simulink model "Cell_model"  (R2024b)
settings: Solver=VariableStepAuto  StartTime=0.0  StopTime=1000  RelTol=1e-3
settings Model: Creator=10537  LastModifiedBy=10537

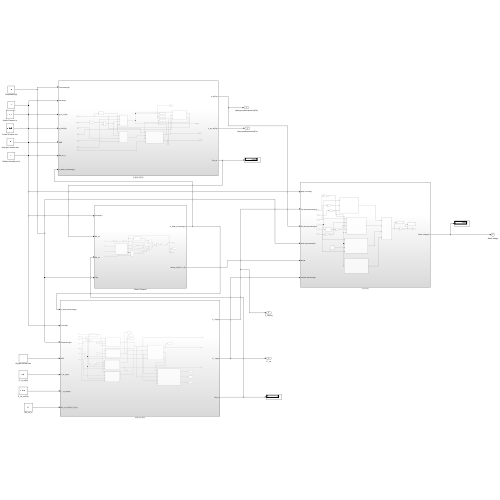
[thumbnail: Simulink's stored preview of the top-level diagram]
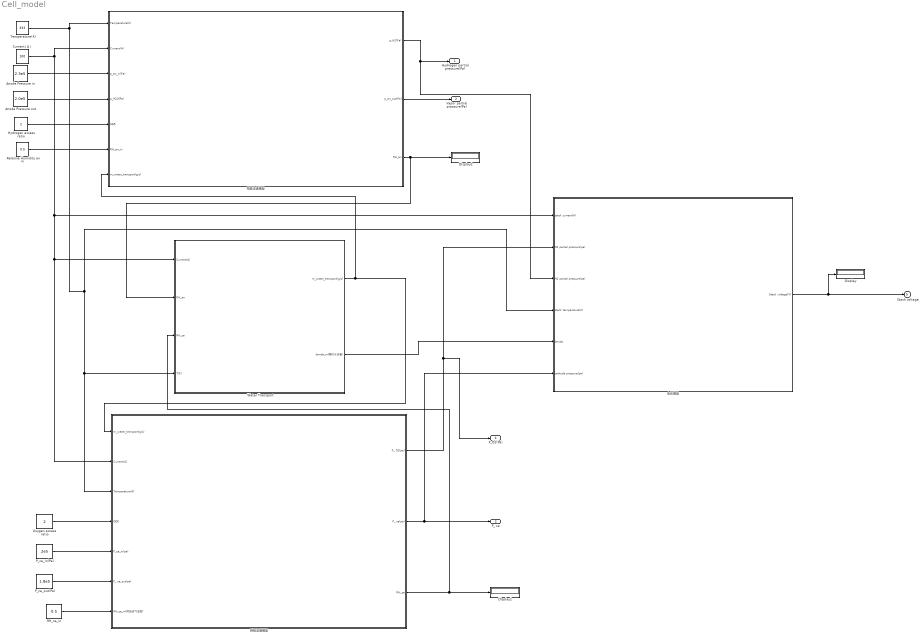
== system Cell_model ==
  " P_ca_in(Pa) " : Constant  Value=2e5
  "Anode Pressure in " : Constant  Value=2.3e5
  "Anode Pressure out " : Constant  Value=2.0e5
  "Current（A） " : Constant  Value=100
  Display : Display
  Display1 : Display
  Display2 : Display
  "Hydrogen excess ratio " : Constant  Value=2
  "Oxygen excess ratio " : Constant  Value=2
  P_ca_out(Pa) : Constant  Value=1.8e5
  RH_ca_in : Constant  Value=0.5
  Relative Humidity an in : Constant  Value=0.5
  Temperature(K) : Constant  Value=333
  Water Transport : Subsystem
  电压模型 : Subsystem
  阳极流道模型 : Subsystem
  阴极流道模型 : Subsystem
  "Hydrogen partial pressure(Pa) " : Outport  VectorParamsAs1DForOutWhenUnconnected=off
  Vapor partial pressure(Pa) : Outport  Port=2  VectorParamsAs1DForOutWhenUnconnected=off
  P_ ca : Outport  Port=3
  P_O2(Pa) : Outport  Port=4
  Stack voltage : Outport  Port=5
  wires:
  Temperature(K)/1 -> 电压模型/4(stack temperature(K)), Water Transport/4(T(K)), 阴极流道模型/3(Temperature(K)), 阳极流道模型/1(Temperature(K))
  "Current（A） "/1 -> Water Transport/1(Current(A)), 阴极流道模型/2(Current(A)), 电压模型/1(stack current(A)), 阳极流道模型/2(Current(A))
  "Anode Pressure in "/1 -> 阳极流道模型/3(p_an_in(Pa))
  "Anode Pressure out "/1 -> 阳极流道模型/4(p_H2O(Pa))
  "Hydrogen excess ratio "/1 -> 阳极流道模型/5(HER)
  Relative Humidity an in/1 -> 阳极流道模型/6(RH_an_in)
  阳极流道模型/1(p_H2(Pa)) -> 电压模型/3(H2 partial pressure(pa)), "Hydrogen partial pressure(Pa) "/1
  阳极流道模型/2(p_an_out(Pa)) -> Vapor partial pressure(Pa)/1
  "Oxygen excess ratio "/1 -> 阴极流道模型/4(OER)
  " P_ca_in(Pa) "/1 -> 阴极流道模型/5(P_ca_in(pa))
  P_ca_out(Pa)/1 -> 阴极流道模型/6(P_ ca_out(pa))
  RH_ca_in/1 -> 阴极流道模型/7(RH_ca_in(阴极进气湿度))
  阴极流道模型/1(P_ O2(pa)) -> 电压模型/2(O2 partial pressure(pa)), P_O2(Pa)/1
  阴极流道模型/2(P_ ca(pa)) -> 电压模型/6(cathode pressure(pa)), P_ ca/1
  电压模型/1(Stack voltage(V)) -> Stack voltage/1, Display/1
  阳极流道模型/3("RH_an ") -> Display2/1, Water Transport/2(RH_an)
  阴极流道模型/3(RH_ca) -> Display1/1, Water Transport/3(RH_ca)
  Water Transport/2(lamda_m(膜的水含量)) -> 电压模型/5(lamda)
  Water Transport/1(m_water_transport(g/s)) -> 阴极流道模型/1(m_water_transport(g/s)), 阳极流道模型/7(m_water_transport(g/s))

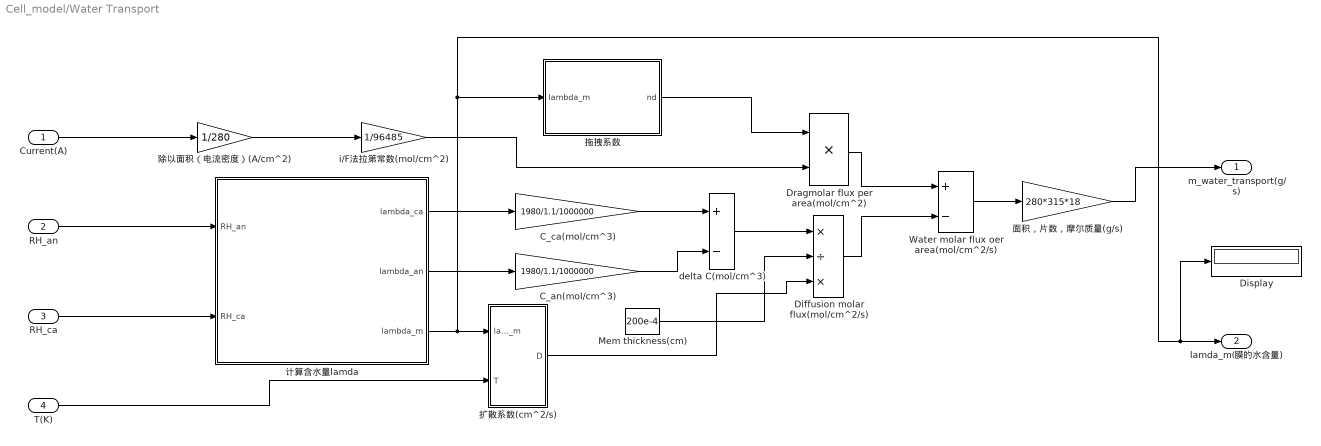
== system Cell_model/Water Transport ==
  Current(A) : Inport
  RH_an : Inport  Port=2
  RH_ca : Inport  Port=3
  T(K) : Inport  Port=4
  "\tC_an(mol/cm^3)" : Gain  Gain=1980/1.1/1000000
  "\tC_ca(mol/cm^3)" : Gain  Gain=1980/1.1/1000000
  Diffusion molar flux(mol/cm^2/s) : Product  Inputs=*/*
  Display : Display
  Dragmolar flux per area(mol/cm^2) : Product
  Mem thickness(cm) : Constant  Value=200e-4
  Water molar flux oer area(mol/cm^2/s) : Sum  Inputs=+-
  delta C(mol/cm^3) : Sum  Inputs=+-
  i/F法拉第常数(mol/cm^2) : Gain  Gain=1/96485
  扩散系数(cm^2/s) : MATLAB Function  TreatAsAtomicUnit=on
  拖拽系数 : MATLAB Function  TreatAsAtomicUnit=on
  计算含水量lamda : MATLAB Function  TreatAsAtomicUnit=on
  除以面积（电流密度）(A/cm^2) : Gain  Gain=1/280
  面积，片数，摩尔质量(g/s) : Gain  Gain=280*315*18
  m_water_transport(g/s) : Outport
  lamda_m(膜的水含量) : Outport  Port=2
  wires:
  除以面积（电流密度）(A/cm^2)/1 -> i/F法拉第常数(mol/cm^2)/1
  计算含水量lamda/1(lambda_ca) -> "\tC_ca(mol/cm^3)"/1
  计算含水量lamda/3(lambda_m) -> lamda_m(膜的水含量)/1, Display/1, 拖拽系数/1(lambda_m), 扩散系数(cm^2/s)/1(lamda_m)
  Diffusion molar flux(mol/cm^2/s)/1 -> Water molar flux oer area(mol/cm^2/s)/2
  Mem thickness(cm)/1 -> Diffusion molar flux(mol/cm^2/s)/2
  扩散系数(cm^2/s)/1(D) -> Diffusion molar flux(mol/cm^2/s)/3
  "\tC_an(mol/cm^3)"/1 -> delta C(mol/cm^3)/2
  Dragmolar flux per area(mol/cm^2)/1 -> Water molar flux oer area(mol/cm^2/s)/1
  Water molar flux oer area(mol/cm^2/s)/1 -> 面积，片数，摩尔质量(g/s)/1
  拖拽系数/1(nd) -> Dragmolar flux per area(mol/cm^2)/1
  i/F法拉第常数(mol/cm^2)/1 -> Dragmolar flux per area(mol/cm^2)/2
  delta C(mol/cm^3)/1 -> Diffusion molar flux(mol/cm^2/s)/1
  计算含水量lamda/2(lambda_an) -> "\tC_an(mol/cm^3)"/1
  "\tC_ca(mol/cm^3)"/1 -> delta C(mol/cm^3)/1
  面积，片数，摩尔质量(g/s)/1 -> m_water_transport(g/s)/1
  T(K)/1 -> 扩散系数(cm^2/s)/2(T)
  Current(A)/1 -> 除以面积（电流密度）(A/cm^2)/1
  RH_an/1 -> 计算含水量lamda/1(RH_an)
  RH_ca/1 -> 计算含水量lamda/2(RH_ca)

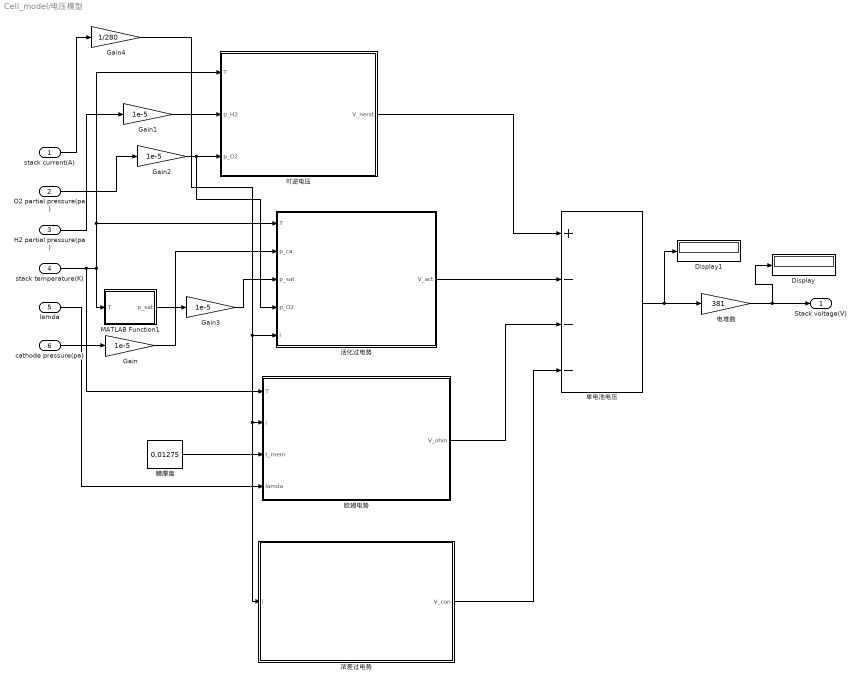
== system Cell_model/电压模型 ==
  stack current(A) : Inport
  O2 partial pressure(pa) : Inport  Port=2
  H2 partial pressure(pa) : Inport  Port=3
  stack temperature(K) : Inport  Port=4
  lamda : Inport  Port=5
  cathode pressure(pa) : Inport  Port=6
  Display : Display
  Display1 : Display
  Gain{,1..3} (4 alike) : Gain  Gain=1e-5
  Gain4 : Gain  Gain=1/280
  MATLAB Function1 : MATLAB Function  TreatAsAtomicUnit=on
  单电池电压 : Sum  Inputs=+---
  可逆电压 : MATLAB Function  TreatAsAtomicUnit=on
  欧姆电势 : MATLAB Function  TreatAsAtomicUnit=on
  活化过电势 : MATLAB Function  TreatAsAtomicUnit=on
  "浓差过电势 " : MATLAB Function  TreatAsAtomicUnit=on
  电堆数 : Gain  Gain=381
  膜厚度 : Constant  Value=0.01275
  Stack voltage(V) : Outport
  wires:
  stack temperature(K)/1 -> 欧姆电势/1(T), MATLAB Function1/1(T), 活化过电势/1(T), 可逆电压/1(T)
  O2 partial pressure(pa)/1 -> Gain2/1
  cathode pressure(pa)/1 -> Gain/1
  H2 partial pressure(pa)/1 -> Gain1/1
  膜厚度/1 -> 欧姆电势/3(t_mem)
  stack current(A)/1 -> Gain4/1
  Gain2/1 -> 活化过电势/4(p_O2), 可逆电压/3(p_O2)
  Gain4/1 -> "浓差过电势 "/1(i), 欧姆电势/2(i), 活化过电势/5(i)
  单电池电压/1 -> Display1/1, 电堆数/1
  MATLAB Function1/1(p_sat) -> Gain3/1
  Gain3/1 -> 活化过电势/3(p_sat)
  "浓差过电势 "/1(V_con) -> 单电池电压/4
  lamda/1 -> 欧姆电势/4(lamda)
  Gain/1 -> 活化过电势/2(p_ca)
  可逆电压/1(V_nerst) -> 单电池电压/1
  电堆数/1 -> Display/1, Stack voltage(V)/1
  活化过电势/1(V_act) -> 单电池电压/2
  Gain1/1 -> 可逆电压/2(p_H2)
  欧姆电势/1(V_ohm) -> 单电池电压/3

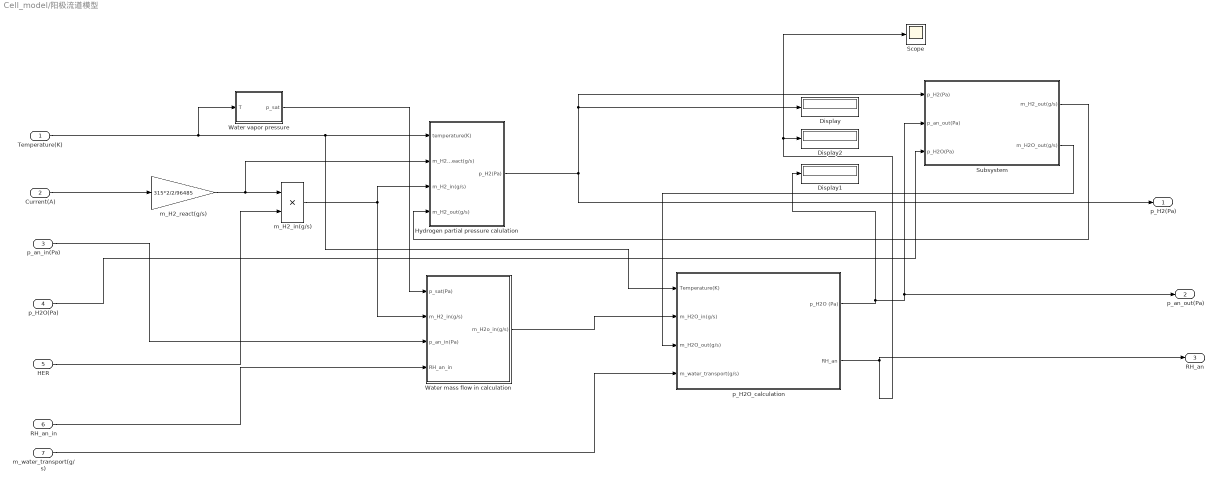
== system Cell_model/阳极流道模型 ==
  Temperature(K) : Inport
  Current(A) : Inport  Port=2
  p_an_in(Pa) : Inport  Port=3
  p_H2O(Pa) : Inport  Port=4
  HER : Inport  Port=5
  RH_an_in : Inport  Port=6
  m_water_transport(g/s) : Inport  Port=7
  Display : Display
  Display1 : Display
  Display2 : Display
  Hydrogen partial pressure calulation : Subsystem
  Scope : Scope
  Subsystem : Subsystem
  Water mass flow in calculation : Subsystem
  Water vapor pressure : MATLAB Function  TreatAsAtomicUnit=on
  m_H2_in(g/s) : Product
  m_H2_react(g/s) : Gain  Gain=315*2/2/96485
  p_H2O_calculation : Subsystem
  p_H2(Pa) : Outport
  p_an_out(Pa) : Outport  Port=2
  "RH_an " : Outport  Port=3
  wires:
  m_H2_in(g/s)/1 -> Water mass flow in calculation/2(m_H2_in(g/s)), Hydrogen partial pressure calulation/3(m_H2_in(g/s))
  Hydrogen partial pressure calulation/1(p_H2(Pa)) -> p_H2(Pa)/1, Display/1, Subsystem/1(p_H2(Pa))
  p_H2O_calculation/1(p_H2O (Pa)) -> Display1/1, p_an_out(Pa)/1, Subsystem/2(p_an_out(Pa))
  HER/1 -> m_H2_in(g/s)/2
  p_H2O_calculation/2("RH_an ") -> "RH_an "/1, Scope/1, Display2/1
  Temperature(K)/1 -> Water vapor pressure/1(T), p_H2O_calculation/1(Temperature(K)), Hydrogen partial pressure calulation/1(temperature(K))
  Subsystem/1(m_H2_out(g/s)) -> Hydrogen partial pressure calulation/4(m_H2_out(g/s))
  Subsystem/2(m_H2O_out(g/s)) -> p_H2O_calculation/3(m_H2O_out(g/s))
  m_H2_react(g/s)/1 -> Hydrogen partial pressure calulation/2(m_H2_react(g/s)), m_H2_in(g/s)/1
  Water mass flow in calculation/1(m_H2o_in(g/s)) -> p_H2O_calculation/2(m_H2O_in(g/s))
  Water vapor pressure/1(p_sat) -> Water mass flow in calculation/1(p_sat(Pa))
  p_H2O(Pa)/1 -> Subsystem/3(p_H2O(Pa))
  Current(A)/1 -> m_H2_react(g/s)/1
  RH_an_in/1 -> Water mass flow in calculation/4(RH_an_in)
  p_an_in(Pa)/1 -> Water mass flow in calculation/3(p_an_in(Pa))
  m_water_transport(g/s)/1 -> p_H2O_calculation/4(m_water_transport(g/s))

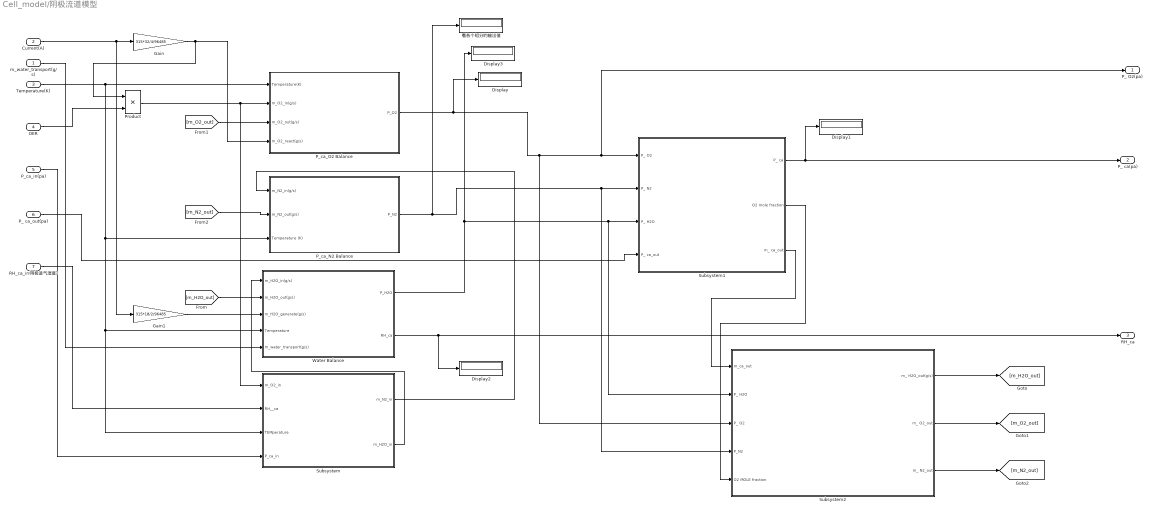
== system Cell_model/阴极流道模型 ==
  m_water_transport(g/s) : Inport
  Current(A) : Inport  Port=2
  Temperature(K) : Inport  Port=3
  OER : Inport  Port=4
  P_ca_in(pa) : Inport  Port=5
  P_ ca_out(pa) : Inport  Port=6
  RH_ca_in(阴极进气湿度) : Inport  Port=7
  Display{,1..3} (4 alike) : Display
  Gain : Gain  Gain=315*32/4/96485
  Gain1 : Gain  Gain=315*18/2/96485
  P_ca_N2 Balance : Subsystem
  P_ca_O2 Balance : Subsystem
  Product : Product
  Subsystem : Subsystem
  Subsystem1 : Subsystem
  Subsystem2 : Subsystem
  Water Balance : Subsystem
  看各个组分的输出值 : Display
  P_ O2(pa) : Outport
  P_ ca(pa) : Outport  Port=2
  RH_ca : Outport  Port=3
  wires:
  [m_H2O_out] -> Water Balance/2(m_H2O_out(g/s))
  Gain1/1 -> Water Balance/3(m_H2O_generate(g/s))
  P_ca_in(pa)/1 -> Subsystem/4(P_ca_in)
  Current(A)/1 -> Gain1/1, Gain/1
  Subsystem2/3(m_ N2_out) -> [m_N2_out]
  P_ca_N2 Balance/1(P_N2) -> 看各个组分的输出值/1, Subsystem2/4(P_N2), Subsystem1/2(P_ N2)
  Water Balance/2(RH_ca) -> RH_ca/1, Display2/1
  Subsystem/2("m_H2O_in ") -> Water Balance/1(m_H2O_in(g/s))
  Subsystem1/1(P_ ca) -> P_ ca(pa)/1, Display1/1
  Temperature(K)/1 -> Subsystem/3(TEMperature), Water Balance/4("Temperature "), P_ca_N2 Balance/3(Temperature (K)), P_ca_O2 Balance/1(Temperature(K))
  Product/1 -> Subsystem/1(m_O2_in), P_ca_O2 Balance/2(m_O2_in(g/s))
  [m_N2_out] -> P_ca_N2 Balance/2(m_N2_out(g/s))
  P_ca_O2 Balance/1(P_O2) -> Display/1, Subsystem2/3(P_ O2), P_ O2(pa)/1, Subsystem1/1(P_ O2)
  Subsystem1/2(O2 mole fraction) -> Subsystem2/5(O2 MOLE fraction)
  Subsystem/1(m_N2_in) -> P_ca_N2 Balance/1(m_N2_in(g/s))
  Subsystem2/2(m_ O2_out) -> [m_O2_out]
  Water Balance/1(P_H2O) -> Subsystem2/2(P_ H2O), Subsystem1/3(P_ H2O), Display3/1
  [m_O2_out] -> P_ca_O2 Balance/3(m_O2_out(g/s))
  P_ ca_out(pa)/1 -> Subsystem1/4(P_ ca_out)
  Gain/1 -> Product/1, P_ca_O2 Balance/4(m_O2_react(g/s))
  Subsystem1/3(m_ ca_out) -> Subsystem2/1(m_ca_out)
  Subsystem2/1(m_ H2O_out(g/s)) -> [m_H2O_out]
  OER/1 -> Product/2
  RH_ca_in(阴极进气湿度)/1 -> Subsystem/2(RH__ca)
  m_water_transport(g/s)/1 -> Water Balance/5(m_water_transport(g/s))

== system Cell_model/阳极流道模型/Hydrogen partial pressure calulation ==
  temperature(K) : Inport
  m_H2_react(g/s) : Inport  Port=2
  m_H2_in(g/s) : Inport  Port=3
  m_H2_out(g/s) : Inport  Port=4
  Gain : Gain  Gain=8.314/2/0.005
  dm_H2/dt(g/s) : Sum  Inputs=+--
  m_H2(g) : Integrator  InitialCondition=0.01
  p_H2 : Product
  p_H2(Pa) : Outport  VectorParamsAs1DForOutWhenUnconnected=off
  wires:
  m_H2_in(g/s)/1 -> dm_H2/dt(g/s)/1
  m_H2(g)/1 -> Gain/1
  m_H2_react(g/s)/1 -> dm_H2/dt(g/s)/2
  Gain/1 -> p_H2/2
  dm_H2/dt(g/s)/1 -> m_H2(g)/1
  p_H2/1 -> p_H2(Pa)/1
  m_H2_out(g/s)/1 -> dm_H2/dt(g/s)/3
  temperature(K)/1 -> p_H2/1

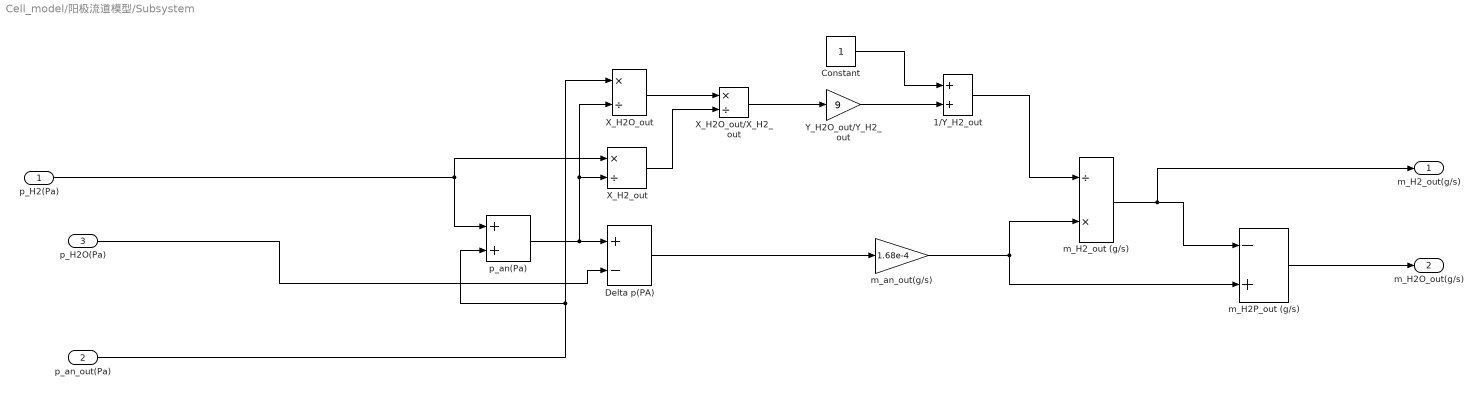
== system Cell_model/阳极流道模型/Subsystem ==
  p_H2(Pa) : Inport
  p_an_out(Pa) : Inport  Port=2
  p_H2O(Pa) : Inport  Port=3
  1/Y_H2_out : Sum
  Constant : Constant
  Delta p(PA) : Sum  Inputs=+-
  X_H2O_out : Product  Inputs=*/
  X_H2O_out/X_H2_out : Product  Inputs=*/
  X_H2_out : Product  Inputs=*/
  Y_H2O_out/Y_H2_out : Gain  Gain=9
  m_H2P_out (g/s) : Sum  Inputs=-+
  m_H2_out (g/s) : Product  Inputs=/*
  m_an_out(g/s) : Gain  Gain=1.68e-4
  p_an(Pa) : Sum
  m_H2_out(g/s) : Outport  VectorParamsAs1DForOutWhenUnconnected=off
  m_H2O_out(g/s) : Outport  Port=2  VectorParamsAs1DForOutWhenUnconnected=off
  wires:
  Delta p(PA)/1 -> m_an_out(g/s)/1
  X_H2O_out/X_H2_out/1 -> Y_H2O_out/Y_H2_out/1
  p_an(Pa)/1 -> X_H2_out/2, X_H2O_out/2, Delta p(PA)/1
  p_H2(Pa)/1 -> p_an(Pa)/1, X_H2_out/1
  m_H2_out (g/s)/1 -> m_H2_out(g/s)/1, m_H2P_out (g/s)/1
  m_an_out(g/s)/1 -> m_H2P_out (g/s)/2, m_H2_out (g/s)/2
  1/Y_H2_out/1 -> m_H2_out (g/s)/1
  p_an_out(Pa)/1 -> p_an(Pa)/2, X_H2O_out/1
  Y_H2O_out/Y_H2_out/1 -> 1/Y_H2_out/2
  Constant/1 -> 1/Y_H2_out/1
  X_H2_out/1 -> X_H2O_out/X_H2_out/2
  X_H2O_out/1 -> X_H2O_out/X_H2_out/1
  m_H2P_out (g/s)/1 -> m_H2O_out(g/s)/1
  p_H2O(Pa)/1 -> Delta p(PA)/2

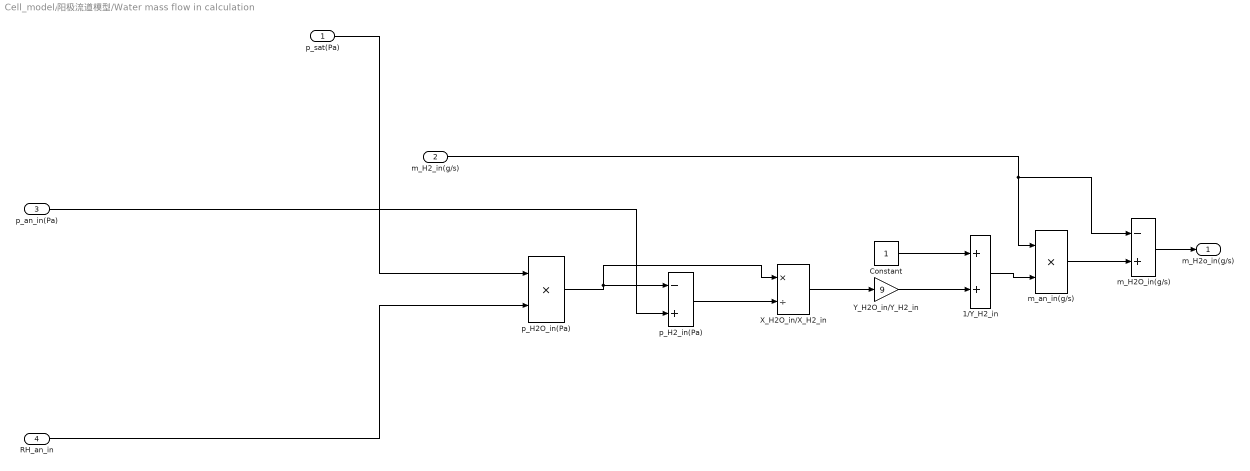
== system Cell_model/阳极流道模型/Water mass flow in calculation ==
  p_sat(Pa) : Inport
  m_H2_in(g/s) : Inport  Port=2
  p_an_in(Pa) : Inport  Port=3
  RH_an_in : Inport  Port=4
  1/Y_H2_in : Sum
  Constant : Constant
  X_H2O_in/X_H2_in : Product  Inputs=*/
  Y_H2O_in/Y_H2_in : Gain  Gain=9
  m_H2O_in(g/s) : Sum  Inputs=-+
  m_an_in(g/s) : Product
  p_H2O_in(Pa) : Product
  p_H2_in(Pa) : Sum  Inputs=-+
  m_H2o_in(g/s) : Outport  VectorParamsAs1DForOutWhenUnconnected=off
  wires:
  1/Y_H2_in/1 -> m_an_in(g/s)/2
  m_an_in(g/s)/1 -> m_H2O_in(g/s)/2
  m_H2_in(g/s)/1 -> m_an_in(g/s)/1, m_H2O_in(g/s)/1
  p_an_in(Pa)/1 -> p_H2_in(Pa)/2
  Y_H2O_in/Y_H2_in/1 -> 1/Y_H2_in/2
  X_H2O_in/X_H2_in/1 -> Y_H2O_in/Y_H2_in/1
  Constant/1 -> 1/Y_H2_in/1
  p_H2_in(Pa)/1 -> X_H2O_in/X_H2_in/2
  p_H2O_in(Pa)/1 -> X_H2O_in/X_H2_in/1, p_H2_in(Pa)/1
  m_H2O_in(g/s)/1 -> m_H2o_in(g/s)/1
  p_sat(Pa)/1 -> p_H2O_in(Pa)/1
  RH_an_in/1 -> p_H2O_in(Pa)/2

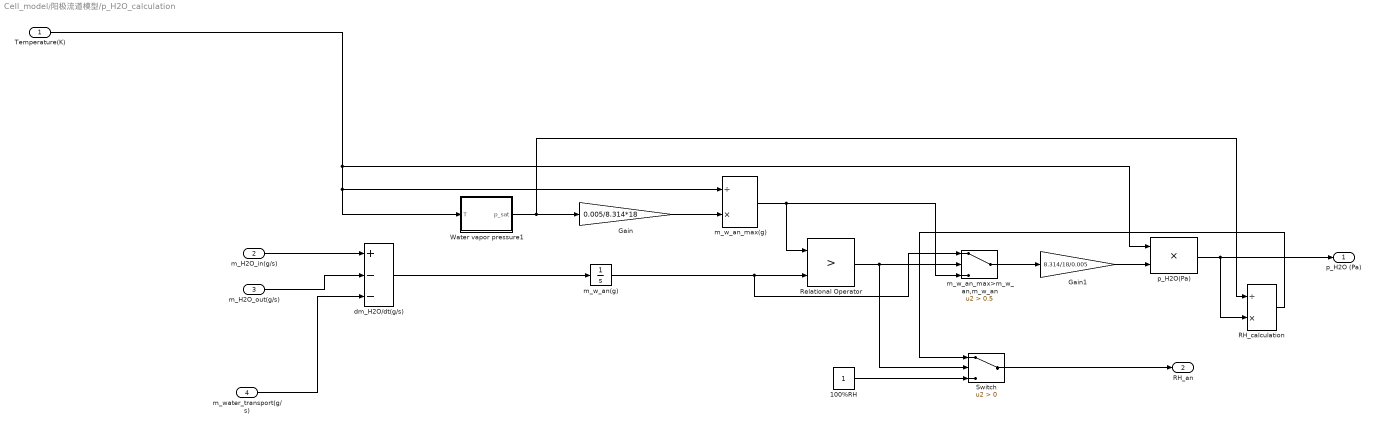
== system Cell_model/阳极流道模型/p_H2O_calculation ==
  Temperature(K) : Inport
  m_H2O_in(g/s) : Inport  Port=2
  m_H2O_out(g/s) : Inport  Port=3
  m_water_transport(g/s) : Inport  Port=4
  100%RH : Constant
  Gain : Gain  Gain=0.005/8.314*18
  Gain1 : Gain  Gain=8.314/18/0.005
  "RH_calculation " : Product  Inputs=/*
  Relational Operator : RelationalOperator  Operator=>  OutDataTypeStr=boolean  RndMeth=Simplest  InputSameDT=off
  Switch : Switch  Criteria=u2 > Threshold  SaturateOnIntegerOverflow=off  InputSameDT=off
  Water vapor pressure1 : MATLAB Function  TreatAsAtomicUnit=on
  dm_H2O/dt(g/s) : Sum  Inputs=+--
  m_w_an(g) : Integrator  InitialCondition=0.01
  m_w_an_max(g) : Product  Inputs=/*
  m_w_an_max>m_w_an,m_w_an : Switch  Criteria=u2 > Threshold  Threshold=0.5  SaturateOnIntegerOverflow=off  InputSameDT=off
  p_H2O(Pa) : Product
  p_H2O (Pa) : Outport  VectorParamsAs1DForOutWhenUnconnected=off
  "RH_an " : Outport  Port=2  VectorParamsAs1DForOutWhenUnconnected=off
  wires:
  Temperature(K)/1 -> Water vapor pressure1/1(T), m_w_an_max(g)/1, p_H2O(Pa)/1
  100%RH/1 -> Switch/3
  m_w_an_max(g)/1 -> m_w_an_max>m_w_an,m_w_an/3, Relational Operator/1
  dm_H2O/dt(g/s)/1 -> m_w_an(g)/1
  Switch/1 -> "RH_an "/1
  m_w_an(g)/1 -> m_w_an_max>m_w_an,m_w_an/1, Relational Operator/2
  Water vapor pressure1/1(p_sat) -> "RH_calculation "/1, Gain/1
  Relational Operator/1 -> Switch/2, m_w_an_max>m_w_an,m_w_an/2
  p_H2O(Pa)/1 -> p_H2O (Pa)/1, "RH_calculation "/2
  Gain1/1 -> p_H2O(Pa)/2
  m_w_an_max>m_w_an,m_w_an/1 -> Gain1/1
  "RH_calculation "/1 -> Switch/1
  Gain/1 -> m_w_an_max(g)/2
  m_H2O_out(g/s)/1 -> dm_H2O/dt(g/s)/2
  m_H2O_in(g/s)/1 -> dm_H2O/dt(g/s)/1
  m_water_transport(g/s)/1 -> dm_H2O/dt(g/s)/3

== system Cell_model/阴极流道模型/P_ca_N2 Balance ==
  m_N2_in(g/s) : Inport
  m_N2_out(g/s) : Inport  Port=2
  Temperature (K) : Inport  Port=3
  Add : Sum  Inputs=+-
  Gain1 : Gain  Gain=8.314/28/0.01
  Product1 : Product
  m_ca_N2 : Integrator  InitialCondition=0.01
  P_N2 : Outport  VectorParamsAs1DForOutWhenUnconnected=off
  wires:
  Add/1 -> m_ca_N2/1
  m_N2_in(g/s)/1 -> Add/1
  m_N2_out(g/s)/1 -> Add/2
  Temperature (K)/1 -> Product1/2
  Gain1/1 -> Product1/1
  Product1/1 -> P_N2/1
  m_ca_N2/1 -> Gain1/1

== system Cell_model/阴极流道模型/P_ca_O2 Balance ==
  Temperature(K) : Inport
  m_O2_in(g/s) : Inport  Port=2
  m_O2_out(g/s) : Inport  Port=3
  m_O2_react(g/s) : Inport  Port=4
  Add : Sum  Inputs=+--
  Gain : Gain  Gain=8.314/32/0.01
  Product : Product
  m_ca_O2 : Integrator  InitialCondition=4.2e4
  P_O2 : Outport  VectorParamsAs1DForOutWhenUnconnected=off
  wires:
  m_O2_react(g/s)/1 -> Add/3
  m_O2_in(g/s)/1 -> Add/1
  Add/1 -> Gain/1
  Temperature(K)/1 -> Product/1
  Gain/1 -> Product/2
  m_O2_out(g/s)/1 -> Add/2
  Product/1 -> m_ca_O2/1
  m_ca_O2/1 -> P_O2/1

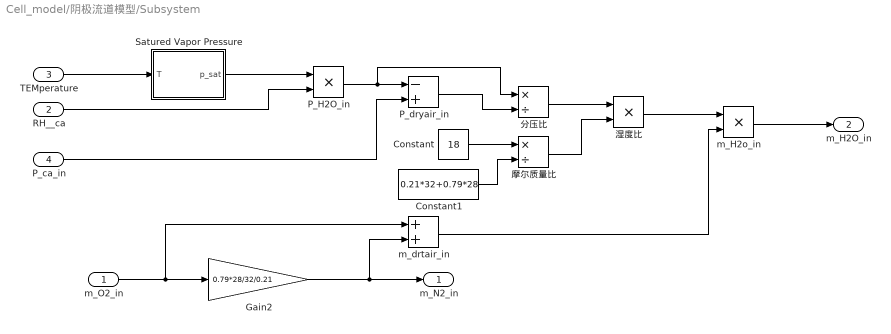
== system Cell_model/阴极流道模型/Subsystem ==
  m_O2_in : Inport
  RH__ca : Inport  Port=2
  TEMperature : Inport  Port=3
  P_ca_in : Inport  Port=4
  Constant : Constant  Value=18
  Constant1 : Constant  Value=0.21*32+0.79*28
  Gain2 : Gain  Gain=0.79*28/32/0.21
  P_H2O_in : Product
  P_dryair_in : Sum  Inputs=-+
  "Satured Vapor Pressure " : MATLAB Function  TreatAsAtomicUnit=on
  "m_H2o_in " : Product
  m_drtair_in : Sum
  分压比 : Product  Inputs=*/
  摩尔质量比 : Product  Inputs=*/
  湿度比 : Product
  m_N2_in : Outport  VectorParamsAs1DForOutWhenUnconnected=off
  "m_H2O_in " : Outport  Port=2  VectorParamsAs1DForOutWhenUnconnected=off
  wires:
  TEMperature/1 -> "Satured Vapor Pressure "/1(T)
  P_ca_in/1 -> P_dryair_in/2
  Gain2/1 -> m_N2_in/1, m_drtair_in/2
  P_H2O_in/1 -> 分压比/1, P_dryair_in/1
  m_O2_in/1 -> m_drtair_in/1, Gain2/1
  Constant1/1 -> 摩尔质量比/2
  摩尔质量比/1 -> 湿度比/2
  湿度比/1 -> "m_H2o_in "/1
  m_drtair_in/1 -> "m_H2o_in "/2
  Constant/1 -> 摩尔质量比/1
  RH__ca/1 -> P_H2O_in/2
  P_dryair_in/1 -> 分压比/2
  "Satured Vapor Pressure "/1(p_sat) -> P_H2O_in/1
  "m_H2o_in "/1 -> "m_H2O_in "/1
  分压比/1 -> 湿度比/1

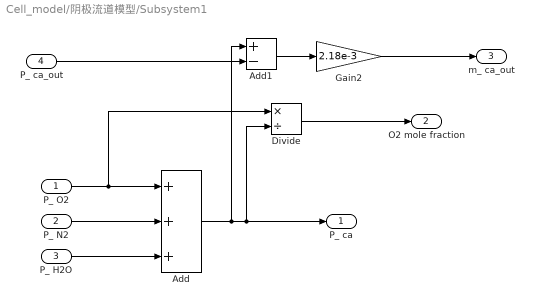
== system Cell_model/阴极流道模型/Subsystem1 ==
  P_ O2 : Inport
  P_ N2 : Inport  Port=2
  P_ H2O : Inport  Port=3
  P_ ca_out : Inport  Port=4
  Add : Sum  Inputs=+++
  Add1 : Sum  Inputs=+-
  Divide : Product  Inputs=*/
  Gain2 : Gain  Gain=2.18e-3
  P_ ca : Outport
  O2 mole fraction : Outport  Port=2
  m_ ca_out : Outport  Port=3
  wires:
  Add1/1 -> Gain2/1
  Add/1 -> Add1/1, P_ ca/1, Divide/2
  P_ H2O/1 -> Add/3
  P_ N2/1 -> Add/2
  P_ ca_out/1 -> Add1/2
  Gain2/1 -> m_ ca_out/1
  P_ O2/1 -> Divide/1, Add/1
  Divide/1 -> O2 mole fraction/1

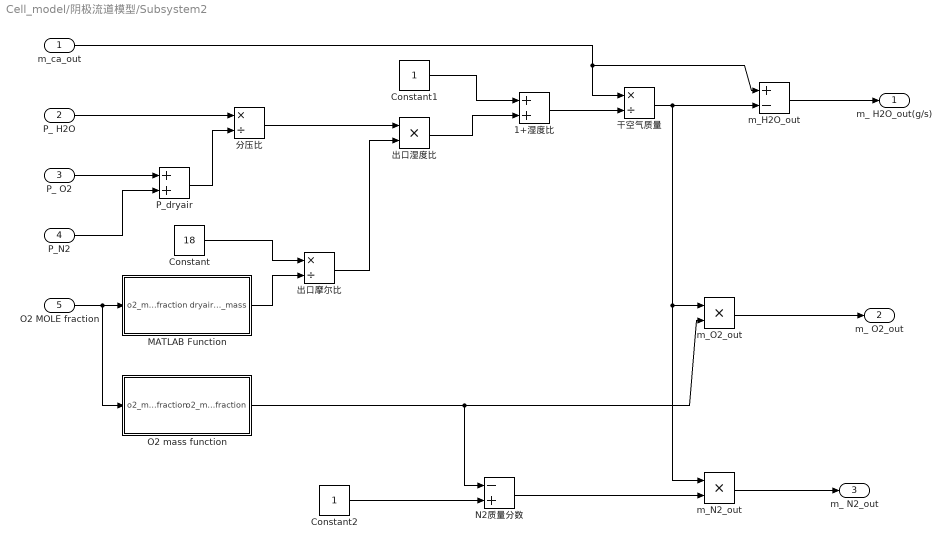
== system Cell_model/阴极流道模型/Subsystem2 ==
  m_ca_out : Inport
  P_ H2O : Inport  Port=2
  P_ O2 : Inport  Port=3
  P_N2 : Inport  Port=4
  O2 MOLE fraction : Inport  Port=5
  1+湿度比 : Sum
  Constant : Constant  Value=18
  Constant1 : Constant
  Constant2 : Constant
  MATLAB Function : MATLAB Function  TreatAsAtomicUnit=on
  N2质量分数 : Sum  Inputs=-+
  O2 mass function : MATLAB Function  TreatAsAtomicUnit=on
  P_dryair : Sum
  m_H2O_out : Sum  Inputs=+-
  m_N2_out : Product
  m_O2_out : Product
  出口摩尔比 : Product  Inputs=*/
  出口湿度比 : Product
  分压比 : Product  Inputs=*/
  干空气质量 : Product  Inputs=*/
  m_ H2O_out(g/s) : Outport
  m_ O2_out : Outport  Port=2
  m_ N2_out : Outport  Port=3
  wires:
  P_dryair/1 -> 分压比/2
  m_ca_out/1 -> m_H2O_out/1, 干空气质量/1
  m_H2O_out/1 -> m_ H2O_out(g/s)/1
  出口摩尔比/1 -> 出口湿度比/2
  出口湿度比/1 -> 1+湿度比/2
  O2 mass function/1(o2_mass_fraction) -> N2质量分数/1, m_O2_out/2
  m_O2_out/1 -> m_ O2_out/1
  干空气质量/1 -> m_H2O_out/2, m_O2_out/1, m_N2_out/1
  P_N2/1 -> P_dryair/2
  N2质量分数/1 -> m_N2_out/2
  P_ O2/1 -> P_dryair/1
  1+湿度比/1 -> 干空气质量/2
  Constant2/1 -> N2质量分数/2
  P_ H2O/1 -> 分压比/1
  分压比/1 -> 出口湿度比/1
  O2 MOLE fraction/1 -> O2 mass function/1(o2_mole_fraction), MATLAB Function/1(o2_mole_fraction)
  MATLAB Function/1(dryair_mole_mass) -> 出口摩尔比/2
  Constant/1 -> 出口摩尔比/1
  Constant1/1 -> 1+湿度比/1
  m_N2_out/1 -> m_ N2_out/1

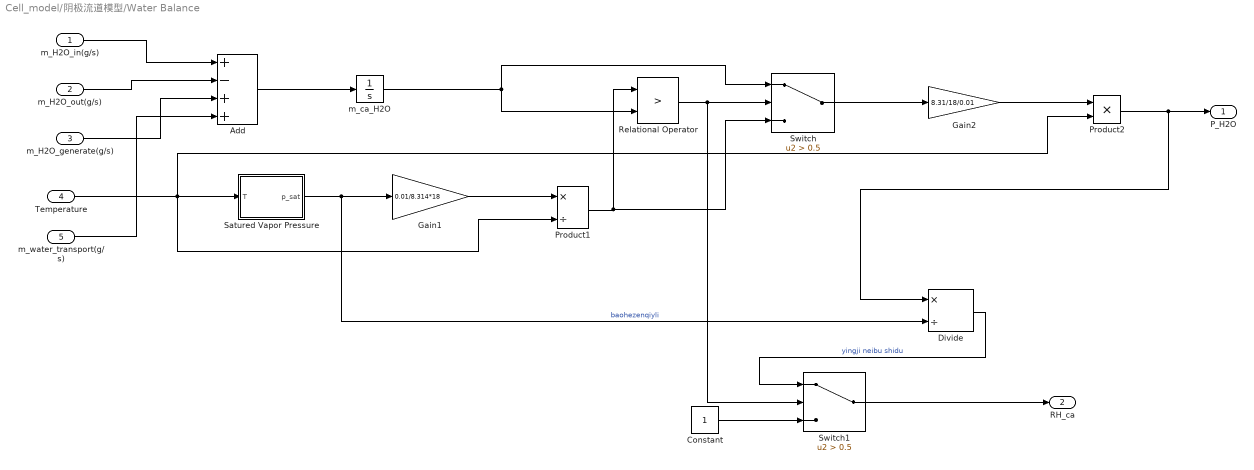
== system Cell_model/阴极流道模型/Water Balance ==
  m_H2O_in(g/s) : Inport
  m_H2O_out(g/s) : Inport  Port=2
  m_H2O_generate(g/s) : Inport  Port=3
  "Temperature " : Inport  Port=4
  m_water_transport(g/s) : Inport  Port=5
  Add : Sum  Inputs=+-++
  Constant : Constant
  Divide : Product  Inputs=*/
  Gain1 : Gain  Gain=0.01/8.314*18
  Gain2 : Gain  Gain=8.31/18/0.01
  Product1 : Product  Inputs=*/
  Product2 : Product
  Relational Operator : RelationalOperator  Operator=>  OutDataTypeStr=boolean  RndMeth=Simplest  InputSameDT=off
  "Satured Vapor Pressure " : MATLAB Function  TreatAsAtomicUnit=on
  Switch : Switch  Criteria=u2 > Threshold  Threshold=0.5  SaturateOnIntegerOverflow=off  InputSameDT=off
  Switch1 : Switch  Criteria=u2 > Threshold  Threshold=0.5  SaturateOnIntegerOverflow=off  InputSameDT=off
  m_ca_H2O : Integrator  InitialCondition=0.01
  P_H2O : Outport  VectorParamsAs1DForOutWhenUnconnected=off
  RH_ca : Outport  Port=2  VectorParamsAs1DForOutWhenUnconnected=off
  wires:
  m_H2O_generate(g/s)/1 -> Add/3
  "Satured Vapor Pressure "/1(p_sat) -> Divide/2, Gain1/1  "baohezenqiyli"
  m_H2O_out(g/s)/1 -> Add/2
  m_ca_H2O/1 -> Relational Operator/2, Switch/1
  Product1/1 -> Switch/3, Relational Operator/1
  Constant/1 -> Switch1/3
  Add/1 -> m_ca_H2O/1
  Switch/1 -> Gain2/1
  Relational Operator/1 -> Switch1/2, Switch/2
  Product2/1 -> P_H2O/1, Divide/1
  Divide/1 -> Switch1/1  "yingji neibu shidu"
  m_H2O_in(g/s)/1 -> Add/1
  Gain1/1 -> Product1/1
  "Temperature "/1 -> Product2/2, Product1/2, "Satured Vapor Pressure "/1(T)
  Switch1/1 -> RH_ca/1
  Gain2/1 -> Product2/1
  m_water_transport(g/s)/1 -> Add/4

== matlab function Cell_model/Water Transport/拖拽系数 ==
  data: lambda_m input; nd output
function nd= fcn(lambda_m)

nd=0.0029*lambda_m^2+0.05/lambda_m-3.4e-19;

== matlab function Cell_model/阳极流道模型/p_H2O_calculation/Water vapor pressure1 ==
  data: T input; p_sat output
function p_sat = fcn(T)%%求水的分压，饱和蒸汽压

p_sat = exp(23.196-3816.44/(T-46.13));

== matlab function Cell_model/Water Transport/计算含水量lamda ==
  data: RH_an input; lambda_ca output; RH_ca input; lambda_an output; lambda_m output
function [lambda_ca,lambda_an,lambda_m]= fcn(RH_an,RH_ca)
if RH_an>=1
    lambda_an=14+1.4*(RH_an-1);
else lambda_an=0.043+17.81*RH_an-39.85*RH_an^2+36*RH_an^3;
end
if RH_ca>=1
    lambda_ca=14+1.4*(RH_ca-1);
else lambda_ca=0.043+17.81*RH_ca-39.85*RH_ca^2+36*RH_ca^3;
end
RH_m = 0.5*(RH_ca+RH_an);
if RH_m>=1
    lambda_m=14+1.4*(RH_m-1);
else lambda_m=0.043+17.81*RH_m-39.85*RH_m^2+36*RH_m^3;
end

== matlab function Cell_model/阳极流道模型/Water vapor pressure ==
  data: T input; p_sat output
function p_sat = fcn(T)%%求水的分压，饱和蒸汽压

p_sat = exp(23.196-3816.44/(T-46.13));

== matlab function Cell_model/阴极流道模型/Subsystem/Satured Vapor Pressure  ==
  data: T input; p_sat output
function p_sat = fcn(T)%%求水的分压，饱和蒸汽压

p_sat = exp(23.196-3816.44/(T-46.13));

== matlab function Cell_model/阴极流道模型/Subsystem2/MATLAB Function ==
  data: o2_mole_fraction input; dryair_mole_mass output
function dryair_mole_mass= fcn(o2_mole_fraction)

dryair_mole_mass = o2_mole_fraction*32+(1-o2_mole_fraction)*28;

== matlab function Cell_model/阴极流道模型/Subsystem2/O2 mass function ==
  data: o2_mole_fraction input; o2_mass_fraction output
function o2_mass_fraction = fcn(o2_mole_fraction)

o2_mass_fraction =(o2_mole_fraction*32) /(o2_mole_fraction*32+(1-o2_mole_fraction)*28);

== matlab function Cell_model/阴极流道模型/Water Balance/Satured Vapor Pressure  ==
  data: T input; p_sat output
function p_sat = fcn(T)%%求水的分压，饱和蒸汽压

p_sat = exp(23.196-3816.44/(T-46.13));

== matlab function Cell_model/电压模型/MATLAB Function1 ==
  data: T input; p_sat output
function p_sat = fcn(T)

p_sat = exp(23.196-3816.44/ (T-46.13));

== matlab function Cell_model/电压模型/可逆电压 ==
  data: T input; V_nerst output; p_H2 input; p_O2 input
function V_nerst= fcn(T,p_H2,p_O2)

V_nerst = 1.229-8.5e-4*(T-298.15)+4.3085e-5*T*(log(p_H2)+0.5*log(p_O2));

== matlab function Cell_model/电压模型/欧姆电势 ==
  data: T input; V_ohm output; i input; t_mem input; lamda input
function V_ohm = fcn(T,i,t_mem,lamda)

sigma=(0.514*lamda-0.033)*exp(1268*(1/303-1/T));
R_ohm=t_mem/sigma;
V_ohm = i*R_ohm;

== matlab function Cell_model/电压模型/活化过电势 ==
  data: T input; V_act output; p_ca input; p_sat input; p_O2 input; i input
function V_act = fcn(T,p_ca,p_sat,p_O2,i)

V0=0.279-8.5e-4*(T-298.15)+4.308e-4*T*(log((p_ca-p_sat)/1.01325)+0.5*log(0.1173*(p_ca-p_sat)/1.01325));
Va = (-1.618e-5*T+1.618e-2)*(p_O2/0.1173+p_sat)^2+(1.8e-4*T-0.166)*(p_O2/0.1173+p_sat)+(-5.8e-4*T+0.5736);
c=10;
V_act = V0+Va*(1-exp(-c*i));

== matlab function Cell_model/电压模型/浓差过电势  ==
  data: i input; V_con output
function V_con = fcn(i)

V_con = 0.016*log(1.5/(1.5-i));

== matlab function Cell_model/Water Transport/扩散系数(cm^2//s) ==
  data: lamda_m input; D output; T input
function D = fcn(lamda_m,T)
if lamda_m<2
    D=1e-6*exp(2416*(1/303-1/T));

elseif lamda_m>=2 && lamda_m<3
    D=1e-6*(1+(2*lamda_m-2))*exp(2416*(1/303-1/T));
elseif lamda_m>=3 && lamda_m<=4.5
    D=1e-6*(3-(1.67*lamda_m-3))*exp(2416*(1/303-1/T));
else 
    D=1.25e-6*exp(2416*(1/303-1/T));
end
